simulink model "graphicalFun1"  (R2017b)
settings: Solver=FixedStepDiscrete  StartTime=0.0  StopTime=10.0  FixedStep=1  RelTol=1e-3
model workspace (MAT data in the model file):
  ContractValidatorBlocksMap = containers.Map
  ContractValidatorBlocksMap.serialization.keys = {'bacteriaPopulationStateflow/bacteriaPopulationSpec/validator', 'bacteriaPopulationStateflow1/bacteriaPopulationSpec/validator', 'bacteriaPopulationTruthTable/bacteriaPopulationSpec/validator', 'truthTable1/bacteriaPopulationSpec/validator', 'truthTable1_PP/bacteriaPopulationSpec/validator'}
  ContractValidatorBlocksMap.serialization.values{1}.block = 'bacteriaPopulationStateflow/bacteriaPopulationSpec/validator'
  ContractValidatorBlocksMap.serialization.values{1}.assumePorts = 1
  ContractValidatorBlocksMap.serialization.values{1}.guaranteePorts = 4
  ContractValidatorBlocksMap.serialization.values{1}.modeBlocksPorts = 3
  ContractValidatorBlocksMap.serialization.values{1}.portHandles.Inport = [317.001098633 318.000366211 319.000366211 320.000366211 321.000366211 322.000366211 323.000366211 324.000366211]
  ContractValidatorBlocksMap.serialization.values{1}.portHandles.Outport = 325.000366211
  ContractValidatorBlocksMap.serialization.values{1}.portHandles.Enable = []
  ContractValidatorBlocksMap.serialization.values{1}.portHandles.Trigger = []
  ContractValidatorBlocksMap.serialization.values{1}.portHandles.State = []
  ContractValidatorBlocksMap.serialization.values{1}.portHandles.LConn = []
  ContractValidatorBlocksMap.serialization.values{1}.portHandles.RConn = []
  ContractValidatorBlocksMap.serialization.values{1}.portHandles.Ifaction = []
  ContractValidatorBlocksMap.serialization.values{1}.portHandles.Reset = []
  ContractValidatorBlocksMap.serialization.values{1}.portConnectivity(1).Type = '1'
  ContractValidatorBlocksMap.serialization.values{1}.portConnectivity(1).Position = [360 -280]
  ContractValidatorBlocksMap.serialization.values{1}.portConnectivity(1).SrcBlock = 21.0003662109
  ContractValidatorBlocksMap.serialization.values{1}.portConnectivity(1).SrcPort = 0
  ContractValidatorBlocksMap.serialization.values{1}.portConnectivity(1).DstBlock = []
  ContractValidatorBlocksMap.serialization.values{1}.portConnectivity(1).DstPort = []
  ContractValidatorBlocksMap.serialization.values{1}.portConnectivity(2).Type = '2'
  ContractValidatorBlocksMap.serialization.values{1}.portConnectivity(2).Position = [360 -170]
  ContractValidatorBlocksMap.serialization.values{1}.portConnectivity(2).SrcBlock = 81.0003662109
  ContractValidatorBlocksMap.serialization.values{1}.portConnectivity(2).SrcPort = 0
  ContractValidatorBlocksMap.serialization.values{1}.portConnectivity(2).DstBlock = []
  ContractValidatorBlocksMap.serialization.values{1}.portConnectivity(2).DstPort = []
  ContractValidatorBlocksMap.serialization.values{1}.portConnectivity(3).Type = '3'
  ContractValidatorBlocksMap.serialization.values{1}.portConnectivity(3).Position = [360 -60]
  ContractValidatorBlocksMap.serialization.values{1}.portConnectivity(3).SrcBlock = 87.0010986328
  ContractValidatorBlocksMap.serialization.values{1}.portConnectivity(3).SrcPort = 0
  ContractValidatorBlocksMap.serialization.values{1}.portConnectivity(3).DstBlock = []
  ContractValidatorBlocksMap.serialization.values{1}.portConnectivity(3).DstPort = []
  ContractValidatorBlocksMap.serialization.values{1}.portConnectivity(4).Type = '4'
  ContractValidatorBlocksMap.serialization.values{1}.portConnectivity(4).Position = [360 50]
  ContractValidatorBlocksMap.serialization.values{1}.portConnectivity(4).SrcBlock = 99.0010986328
  ContractValidatorBlocksMap.serialization.values{1}.portConnectivity(4).SrcPort = 0
  ContractValidatorBlocksMap.serialization.values{1}.portConnectivity(4).DstBlock = []
  ContractValidatorBlocksMap.serialization.values{1}.portConnectivity(4).DstPort = []
  ContractValidatorBlocksMap.serialization.values{1}.portConnectivity(5).Type = '5'
  ContractValidatorBlocksMap.serialization.values{1}.portConnectivity(5).Position = [360 160]
  ContractValidatorBlocksMap.serialization.values{1}.portConnectivity(5).SrcBlock = 148.001098633
  ContractValidatorBlocksMap.serialization.values{1}.portConnectivity(5).SrcPort = 0
  ContractValidatorBlocksMap.serialization.values{1}.portConnectivity(5).DstBlock = []
  ContractValidatorBlocksMap.serialization.values{1}.portConnectivity(5).DstPort = []
  ContractValidatorBlocksMap.serialization.values{1}.portConnectivity(6).Type = '6'
  ContractValidatorBlocksMap.serialization.values{1}.portConnectivity(6).Position = [360 270]
  ContractValidatorBlocksMap.serialization.values{1}.portConnectivity(6).SrcBlock = 197.001098633
  ContractValidatorBlocksMap.serialization.values{1}.portConnectivity(6).SrcPort = 0
  ContractValidatorBlocksMap.serialization.values{1}.portConnectivity(6).DstBlock = []
  ContractValidatorBlocksMap.serialization.values{1}.portConnectivity(6).DstPort = []
  ContractValidatorBlocksMap.serialization.values{1}.portConnectivity(7).Type = '7'
  ContractValidatorBlocksMap.serialization.values{1}.portConnectivity(7).Position = [360 380]
  ContractValidatorBlocksMap.serialization.values{1}.portConnectivity(7).SrcBlock = 27.0010986328
  ContractValidatorBlocksMap.serialization.values{1}.portConnectivity(7).SrcPort = 0
  ContractValidatorBlocksMap.serialization.values{1}.portConnectivity(7).DstBlock = []
  ContractValidatorBlocksMap.serialization.values{1}.portConnectivity(7).DstPort = []
  ContractValidatorBlocksMap.serialization.values{1}.portConnectivity(8).Type = '8'
  ContractValidatorBlocksMap.serialization.values{1}.portConnectivity(8).Position = [360 490]
  ContractValidatorBlocksMap.serialization.values{1}.portConnectivity(8).SrcBlock = 238.001098633
  ContractValidatorBlocksMap.serialization.values{1}.portConnectivity(8).SrcPort = 0
  ContractValidatorBlocksMap.serialization.values{1}.portConnectivity(8).DstBlock = []
  ContractValidatorBlocksMap.serialization.values{1}.portConnectivity(8).DstPort = []
  ContractValidatorBlocksMap.serialization.values{1}.portConnectivity(9).Type = '1'
  ContractValidatorBlocksMap.serialization.values{1}.portConnectivity(9).Position = [500 105]
  ContractValidatorBlocksMap.serialization.values{1}.portConnectivity(9).SrcBlock = []
  ContractValidatorBlocksMap.serialization.values{1}.portConnectivity(9).SrcPort = []
  ContractValidatorBlocksMap.serialization.values{1}.portConnectivity(9).DstBlock = [250.000366211 20.0003662109]
  ContractValidatorBlocksMap.serialization.values{1}.portConnectivity(9).DstPort = [0 0]
  ContractValidatorBlocksMap.serialization.values{2}.block = 'bacteriaPopulationStateflow1/bacteriaPopulationSpec/validator'
  ContractValidatorBlocksMap.serialization.values{2}.assumePorts = 1
  ContractValidatorBlocksMap.serialization.values{2}.guaranteePorts = 4
  ContractValidatorBlocksMap.serialization.values{2}.modeBlocksPorts = 3
  ContractValidatorBlocksMap.serialization.values{2}.portHandles.Inport = [309.001586914 310.001220703 311.000854492 312.000976562 313.000976562 314.001098633 315.000976562 316.000854492]
  ContractValidatorBlocksMap.serialization.values{2}.portHandles.Outport = 317.001098633
  ContractValidatorBlocksMap.serialization.values{2}.portHandles.Enable = []
  ContractValidatorBlocksMap.serialization.values{2}.portHandles.Trigger = []
  ContractValidatorBlocksMap.serialization.values{2}.portHandles.State = []
  ContractValidatorBlocksMap.serialization.values{2}.portHandles.LConn = []
  ContractValidatorBlocksMap.serialization.values{2}.portHandles.RConn = []
  ContractValidatorBlocksMap.serialization.values{2}.portHandles.Ifaction = []
  ContractValidatorBlocksMap.serialization.values{2}.portHandles.Reset = []
  ContractValidatorBlocksMap.serialization.values{2}.portConnectivity(1).Type = '1'
  ContractValidatorBlocksMap.serialization.values{2}.portConnectivity(1).Position = [360 -280]
  ContractValidatorBlocksMap.serialization.values{2}.portConnectivity(1).SrcBlock = 21.0007324219
  ContractValidatorBlocksMap.serialization.values{2}.portConnectivity(1).SrcPort = 0
  ContractValidatorBlocksMap.serialization.values{2}.portConnectivity(1).DstBlock = []
  ContractValidatorBlocksMap.serialization.values{2}.portConnectivity(1).DstPort = []
  ContractValidatorBlocksMap.serialization.values{2}.portConnectivity(2).Type = '2'
  ContractValidatorBlocksMap.serialization.values{2}.portConnectivity(2).Position = [360 -170]
  ContractValidatorBlocksMap.serialization.values{2}.portConnectivity(2).SrcBlock = 81.0010986328
  ContractValidatorBlocksMap.serialization.values{2}.portConnectivity(2).SrcPort = 0
  ContractValidatorBlocksMap.serialization.values{2}.portConnectivity(2).DstBlock = []
  ContractValidatorBlocksMap.serialization.values{2}.portConnectivity(2).DstPort = []
  ContractValidatorBlocksMap.serialization.values{2}.portConnectivity(3).Type = '3'
  ContractValidatorBlocksMap.serialization.values{2}.portConnectivity(3).Position = [360 -60]
  ContractValidatorBlocksMap.serialization.values{2}.portConnectivity(3).SrcBlock = 87.0009765625
  ContractValidatorBlocksMap.serialization.values{2}.portConnectivity(3).SrcPort = 0
  ContractValidatorBlocksMap.serialization.values{2}.portConnectivity(3).DstBlock = []
  ContractValidatorBlocksMap.serialization.values{2}.portConnectivity(3).DstPort = []
  ContractValidatorBlocksMap.serialization.values{2}.portConnectivity(4).Type = '4'
  ContractValidatorBlocksMap.serialization.values{2}.portConnectivity(4).Position = [360 50]
  ContractValidatorBlocksMap.serialization.values{2}.portConnectivity(4).SrcBlock = 99.0009765625
  ContractValidatorBlocksMap.serialization.values{2}.portConnectivity(4).SrcPort = 0
  ContractValidatorBlocksMap.serialization.values{2}.portConnectivity(4).DstBlock = []
  ContractValidatorBlocksMap.serialization.values{2}.portConnectivity(4).DstPort = []
  ContractValidatorBlocksMap.serialization.values{2}.portConnectivity(5).Type = '5'
  ContractValidatorBlocksMap.serialization.values{2}.portConnectivity(5).Position = [360 160]
  ContractValidatorBlocksMap.serialization.values{2}.portConnectivity(5).SrcBlock = 148.000976562
  ContractValidatorBlocksMap.serialization.values{2}.portConnectivity(5).SrcPort = 0
  ContractValidatorBlocksMap.serialization.values{2}.portConnectivity(5).DstBlock = []
  ContractValidatorBlocksMap.serialization.values{2}.portConnectivity(5).DstPort = []
  ContractValidatorBlocksMap.serialization.values{2}.portConnectivity(6).Type = '6'
  ContractValidatorBlocksMap.serialization.values{2}.portConnectivity(6).Position = [360 270]
  ContractValidatorBlocksMap.serialization.values{2}.portConnectivity(6).SrcBlock = 197.000976562
  ContractValidatorBlocksMap.serialization.values{2}.portConnectivity(6).SrcPort = 0
  ContractValidatorBlocksMap.serialization.values{2}.portConnectivity(6).DstBlock = []
  ContractValidatorBlocksMap.serialization.values{2}.portConnectivity(6).DstPort = []
  ContractValidatorBlocksMap.serialization.values{2}.portConnectivity(7).Type = '7'
  ContractValidatorBlocksMap.serialization.values{2}.portConnectivity(7).Position = [360 380]
  ContractValidatorBlocksMap.serialization.values{2}.portConnectivity(7).SrcBlock = 27.0018310547
  ContractValidatorBlocksMap.serialization.values{2}.portConnectivity(7).SrcPort = 0
  ContractValidatorBlocksMap.serialization.values{2}.portConnectivity(7).DstBlock = []
  ContractValidatorBlocksMap.serialization.values{2}.portConnectivity(7).DstPort = []
  ContractValidatorBlocksMap.serialization.values{2}.portConnectivity(8).Type = '8'
  ContractValidatorBlocksMap.serialization.values{2}.portConnectivity(8).Position = [360 490]
  ContractValidatorBlocksMap.serialization.values{2}.portConnectivity(8).SrcBlock = 238.000976562
  ContractValidatorBlocksMap.serialization.values{2}.portConnectivity(8).SrcPort = 0
  ContractValidatorBlocksMap.serialization.values{2}.portConnectivity(8).DstBlock = []
  ContractValidatorBlocksMap.serialization.values{2}.portConnectivity(8).DstPort = []
  ContractValidatorBlocksMap.serialization.values{2}.portConnectivity(9).Type = '1'
  ContractValidatorBlocksMap.serialization.values{2}.portConnectivity(9).Position = [500 105]
  ContractValidatorBlocksMap.serialization.values{2}.portConnectivity(9).SrcBlock = []
  ContractValidatorBlocksMap.serialization.values{2}.portConnectivity(9).SrcPort = []
  ContractValidatorBlocksMap.serialization.values{2}.portConnectivity(9).DstBlock = [250.000488281 20.0009765625]
  ContractValidatorBlocksMap.serialization.values{2}.portConnectivity(9).DstPort = [0 0]
  ContractValidatorBlocksMap.serialization.values{3}.block = 'bacteriaPopulationTruthTable/bacteriaPopulationSpec/validator'
  ContractValidatorBlocksMap.serialization.values{3}.assumePorts = 1
  ContractValidatorBlocksMap.serialization.values{3}.guaranteePorts = 4
  ContractValidatorBlocksMap.serialization.values{3}.modeBlocksPorts = 3
  ContractValidatorBlocksMap.serialization.values{3}.portHandles.Inport = [317.001831055 318.001342773 319.001342773 320.001342773 321.001342773 322.001342773 323.001342773 324.001342773]
  ContractValidatorBlocksMap.serialization.values{3}.portHandles.Outport = 325.000976562
  ContractValidatorBlocksMap.serialization.values{3}.portHandles.Enable = []
  ContractValidatorBlocksMap.serialization.values{3}.portHandles.Trigger = []
  ContractValidatorBlocksMap.serialization.values{3}.portHandles.State = []
  ContractValidatorBlocksMap.serialization.values{3}.portHandles.LConn = []
  ContractValidatorBlocksMap.serialization.values{3}.portHandles.RConn = []
  ContractValidatorBlocksMap.serialization.values{3}.portHandles.Ifaction = []
  ContractValidatorBlocksMap.serialization.values{3}.portHandles.Reset = []
  ContractValidatorBlocksMap.serialization.values{3}.portConnectivity(1).Type = '1'
  ContractValidatorBlocksMap.serialization.values{3}.portConnectivity(1).Position = [360 -280]
  ContractValidatorBlocksMap.serialization.values{3}.portConnectivity(1).SrcBlock = 21.0007324219
  ContractValidatorBlocksMap.serialization.values{3}.portConnectivity(1).SrcPort = 0
  ContractValidatorBlocksMap.serialization.values{3}.portConnectivity(1).DstBlock = []
  ContractValidatorBlocksMap.serialization.values{3}.portConnectivity(1).DstPort = []
  ContractValidatorBlocksMap.serialization.values{3}.portConnectivity(2).Type = '2'
  ContractValidatorBlocksMap.serialization.values{3}.portConnectivity(2).Position = [360 -170]
  ContractValidatorBlocksMap.serialization.values{3}.portConnectivity(2).SrcBlock = 81.0007324219
  ContractValidatorBlocksMap.serialization.values{3}.portConnectivity(2).SrcPort = 0
  ContractValidatorBlocksMap.serialization.values{3}.portConnectivity(2).DstBlock = []
  ContractValidatorBlocksMap.serialization.values{3}.portConnectivity(2).DstPort = []
  ContractValidatorBlocksMap.serialization.values{3}.portConnectivity(3).Type = '3'
  ContractValidatorBlocksMap.serialization.values{3}.portConnectivity(3).Position = [360 -60]
  ContractValidatorBlocksMap.serialization.values{3}.portConnectivity(3).SrcBlock = 87.0012207031
  ContractValidatorBlocksMap.serialization.values{3}.portConnectivity(3).SrcPort = 0
  ContractValidatorBlocksMap.serialization.values{3}.portConnectivity(3).DstBlock = []
  ContractValidatorBlocksMap.serialization.values{3}.portConnectivity(3).DstPort = []
  ContractValidatorBlocksMap.serialization.values{3}.portConnectivity(4).Type = '4'
  ContractValidatorBlocksMap.serialization.values{3}.portConnectivity(4).Position = [360 50]
  ContractValidatorBlocksMap.serialization.values{3}.portConnectivity(4).SrcBlock = 99.0014648438
  ContractValidatorBlocksMap.serialization.values{3}.portConnectivity(4).SrcPort = 0
  ContractValidatorBlocksMap.serialization.values{3}.portConnectivity(4).DstBlock = []
  ContractValidatorBlocksMap.serialization.values{3}.portConnectivity(4).DstPort = []
  ContractValidatorBlocksMap.serialization.values{3}.portConnectivity(5).Type = '5'
  ContractValidatorBlocksMap.serialization.values{3}.portConnectivity(5).Position = [360 160]
  ContractValidatorBlocksMap.serialization.values{3}.portConnectivity(5).SrcBlock = 148.001220703
  ContractValidatorBlocksMap.serialization.values{3}.portConnectivity(5).SrcPort = 0
  ContractValidatorBlocksMap.serialization.values{3}.portConnectivity(5).DstBlock = []
  ContractValidatorBlocksMap.serialization.values{3}.portConnectivity(5).DstPort = []
  ContractValidatorBlocksMap.serialization.values{3}.portConnectivity(6).Type = '6'
  ContractValidatorBlocksMap.serialization.values{3}.portConnectivity(6).Position = [360 270]
  ContractValidatorBlocksMap.serialization.values{3}.portConnectivity(6).SrcBlock = 197.001098633
  ContractValidatorBlocksMap.serialization.values{3}.portConnectivity(6).SrcPort = 0
  ContractValidatorBlocksMap.serialization.values{3}.portConnectivity(6).DstBlock = []
  ContractValidatorBlocksMap.serialization.values{3}.portConnectivity(6).DstPort = []
  ContractValidatorBlocksMap.serialization.values{3}.portConnectivity(7).Type = '7'
  ContractValidatorBlocksMap.serialization.values{3}.portConnectivity(7).Position = [360 380]
  ContractValidatorBlocksMap.serialization.values{3}.portConnectivity(7).SrcBlock = 27.0021972656
  ContractValidatorBlocksMap.serialization.values{3}.portConnectivity(7).SrcPort = 0
  ContractValidatorBlocksMap.serialization.values{3}.portConnectivity(7).DstBlock = []
  ContractValidatorBlocksMap.serialization.values{3}.portConnectivity(7).DstPort = []
  ContractValidatorBlocksMap.serialization.values{3}.portConnectivity(8).Type = '8'
  ContractValidatorBlocksMap.serialization.values{3}.portConnectivity(8).Position = [360 490]
  ContractValidatorBlocksMap.serialization.values{3}.portConnectivity(8).SrcBlock = 238.001098633
  ContractValidatorBlocksMap.serialization.values{3}.portConnectivity(8).SrcPort = 0
  ContractValidatorBlocksMap.serialization.values{3}.portConnectivity(8).DstBlock = []
  ContractValidatorBlocksMap.serialization.values{3}.portConnectivity(8).DstPort = []
  ContractValidatorBlocksMap.serialization.values{3}.portConnectivity(9).Type = '1'
  ContractValidatorBlocksMap.serialization.values{3}.portConnectivity(9).Position = [500 105]
  ContractValidatorBlocksMap.serialization.values{3}.portConnectivity(9).SrcBlock = []
  ContractValidatorBlocksMap.serialization.values{3}.portConnectivity(9).SrcPort = []
  ContractValidatorBlocksMap.serialization.values{3}.portConnectivity(9).DstBlock = [250.000610352 20.0007324219]
  ContractValidatorBlocksMap.serialization.values{3}.portConnectivity(9).DstPort = [0 0]
  ContractValidatorBlocksMap.serialization.values{4}.block = 'truthTable1/bacteriaPopulationSpec/validator'
  ContractValidatorBlocksMap.serialization.values{4}.assumePorts = 1
  ContractValidatorBlocksMap.serialization.values{4}.guaranteePorts = 4
  ContractValidatorBlocksMap.serialization.values{4}.modeBlocksPorts = 3
  ContractValidatorBlocksMap.serialization.values{4}.portHandles.Inport = [317.000732422 318.000244141 319.000244141 320.000244141 321.000244141 322.000244141 323.000244141 324.000244141]
  ContractValidatorBlocksMap.serialization.values{4}.portHandles.Outport = 325.000244141
  ContractValidatorBlocksMap.serialization.values{4}.portHandles.Enable = []
  ContractValidatorBlocksMap.serialization.values{4}.portHandles.Trigger = []
  ContractValidatorBlocksMap.serialization.values{4}.portHandles.State = []
  ContractValidatorBlocksMap.serialization.values{4}.portHandles.LConn = []
  ContractValidatorBlocksMap.serialization.values{4}.portHandles.RConn = []
  ContractValidatorBlocksMap.serialization.values{4}.portHandles.Ifaction = []
  ContractValidatorBlocksMap.serialization.values{4}.portHandles.Reset = []
  ContractValidatorBlocksMap.serialization.values{4}.portConnectivity(1).Type = '1'
  ContractValidatorBlocksMap.serialization.values{4}.portConnectivity(1).Position = [360 -280]
  ContractValidatorBlocksMap.serialization.values{4}.portConnectivity(1).SrcBlock = 21.0002441406
  ContractValidatorBlocksMap.serialization.values{4}.portConnectivity(1).SrcPort = 0
  ContractValidatorBlocksMap.serialization.values{4}.portConnectivity(1).DstBlock = []
  ContractValidatorBlocksMap.serialization.values{4}.portConnectivity(1).DstPort = []
  ContractValidatorBlocksMap.serialization.values{4}.portConnectivity(2).Type = '2'
  ContractValidatorBlocksMap.serialization.values{4}.portConnectivity(2).Position = [360 -170]
  ContractValidatorBlocksMap.serialization.values{4}.portConnectivity(2).SrcBlock = 81.0002441406
  ContractValidatorBlocksMap.serialization.values{4}.portConnectivity(2).SrcPort = 0
  ContractValidatorBlocksMap.serialization.values{4}.portConnectivity(2).DstBlock = []
  ContractValidatorBlocksMap.serialization.values{4}.portConnectivity(2).DstPort = []
  ContractValidatorBlocksMap.serialization.values{4}.portConnectivity(3).Type = '3'
  ContractValidatorBlocksMap.serialization.values{4}.portConnectivity(3).Position = [360 -60]
  ContractValidatorBlocksMap.serialization.values{4}.portConnectivity(3).SrcBlock = 87.0007324219
  ContractValidatorBlocksMap.serialization.values{4}.portConnectivity(3).SrcPort = 0
  ContractValidatorBlocksMap.serialization.values{4}.portConnectivity(3).DstBlock = []
  ContractValidatorBlocksMap.serialization.values{4}.portConnectivity(3).DstPort = []
  ContractValidatorBlocksMap.serialization.values{4}.portConnectivity(4).Type = '4'
  ContractValidatorBlocksMap.serialization.values{4}.portConnectivity(4).Position = [360 50]
  ContractValidatorBlocksMap.serialization.values{4}.portConnectivity(4).SrcBlock = 99.0007324219
  ContractValidatorBlocksMap.serialization.values{4}.portConnectivity(4).SrcPort = 0
  ContractValidatorBlocksMap.serialization.values{4}.portConnectivity(4).DstBlock = []
  ContractValidatorBlocksMap.serialization.values{4}.portConnectivity(4).DstPort = []
  ContractValidatorBlocksMap.serialization.values{4}.portConnectivity(5).Type = '5'
  ContractValidatorBlocksMap.serialization.values{4}.portConnectivity(5).Position = [360 160]
  ContractValidatorBlocksMap.serialization.values{4}.portConnectivity(5).SrcBlock = 148.000732422
  ContractValidatorBlocksMap.serialization.values{4}.portConnectivity(5).SrcPort = 0
  ContractValidatorBlocksMap.serialization.values{4}.portConnectivity(5).DstBlock = []
  ContractValidatorBlocksMap.serialization.values{4}.portConnectivity(5).DstPort = []
  ContractValidatorBlocksMap.serialization.values{4}.portConnectivity(6).Type = '6'
  ContractValidatorBlocksMap.serialization.values{4}.portConnectivity(6).Position = [360 270]
  ContractValidatorBlocksMap.serialization.values{4}.portConnectivity(6).SrcBlock = 197.000732422
  ContractValidatorBlocksMap.serialization.values{4}.portConnectivity(6).SrcPort = 0
  ContractValidatorBlocksMap.serialization.values{4}.portConnectivity(6).DstBlock = []
  ContractValidatorBlocksMap.serialization.values{4}.portConnectivity(6).DstPort = []
  ContractValidatorBlocksMap.serialization.values{4}.portConnectivity(7).Type = '7'
  ContractValidatorBlocksMap.serialization.values{4}.portConnectivity(7).Position = [360 380]
  ContractValidatorBlocksMap.serialization.values{4}.portConnectivity(7).SrcBlock = 27.0007324219
  ContractValidatorBlocksMap.serialization.values{4}.portConnectivity(7).SrcPort = 0
  ContractValidatorBlocksMap.serialization.values{4}.portConnectivity(7).DstBlock = []
  ContractValidatorBlocksMap.serialization.values{4}.portConnectivity(7).DstPort = []
  ContractValidatorBlocksMap.serialization.values{4}.portConnectivity(8).Type = '8'
  ContractValidatorBlocksMap.serialization.values{4}.portConnectivity(8).Position = [360 490]
  ContractValidatorBlocksMap.serialization.values{4}.portConnectivity(8).SrcBlock = 238.000732422
  ContractValidatorBlocksMap.serialization.values{4}.portConnectivity(8).SrcPort = 0
  ContractValidatorBlocksMap.serialization.values{4}.portConnectivity(8).DstBlock = []
  ContractValidatorBlocksMap.serialization.values{4}.portConnectivity(8).DstPort = []
  ContractValidatorBlocksMap.serialization.values{4}.portConnectivity(9).Type = '1'
  ContractValidatorBlocksMap.serialization.values{4}.portConnectivity(9).Position = [500 105]
  ContractValidatorBlocksMap.serialization.values{4}.portConnectivity(9).SrcBlock = []
  ContractValidatorBlocksMap.serialization.values{4}.portConnectivity(9).SrcPort = []
  ContractValidatorBlocksMap.serialization.values{4}.portConnectivity(9).DstBlock = [250.000244141 20.0002441406]
  ContractValidatorBlocksMap.serialization.values{4}.portConnectivity(9).DstPort = [0 0]
  ContractValidatorBlocksMap.serialization.values{5}.block = 'truthTable1_PP/bacteriaPopulationSpec/validator'
  ContractValidatorBlocksMap.serialization.values{5}.assumePorts = 1
  ContractValidatorBlocksMap.serialization.values{5}.guaranteePorts = 4
  ContractValidatorBlocksMap.serialization.values{5}.modeBlocksPorts = 3
  ContractValidatorBlocksMap.serialization.values{5}.portHandles.Inport = [1295.00036621 1296.00012207 1297.00012207 1298.00012207 1299.00012207 1300.00012207 1301.00012207 1302.00012207]
  ContractValidatorBlocksMap.serialization.values{5}.portHandles.Outport = 1303.00012207
  ContractValidatorBlocksMap.serialization.values{5}.portHandles.Enable = []
  ContractValidatorBlocksMap.serialization.values{5}.portHandles.Trigger = []
  ContractValidatorBlocksMap.serialization.values{5}.portHandles.State = []
  ContractValidatorBlocksMap.serialization.values{5}.portHandles.LConn = []
  ContractValidatorBlocksMap.serialization.values{5}.portHandles.RConn = []
  ContractValidatorBlocksMap.serialization.values{5}.portHandles.Ifaction = []
  ContractValidatorBlocksMap.serialization.values{5}.portHandles.Reset = []
  ContractValidatorBlocksMap.serialization.values{5}.portConnectivity(1).Type = '1'
  ContractValidatorBlocksMap.serialization.values{5}.portConnectivity(1).Position = [360 -280]
  ContractValidatorBlocksMap.serialization.values{5}.portConnectivity(1).SrcBlock = 350.000488281
  ContractValidatorBlocksMap.serialization.values{5}.portConnectivity(1).SrcPort = 0
  ContractValidatorBlocksMap.serialization.values{5}.portConnectivity(1).DstBlock = []
  ContractValidatorBlocksMap.serialization.values{5}.portConnectivity(1).DstPort = []
  ContractValidatorBlocksMap.serialization.values{5}.portConnectivity(2).Type = '2'
  ContractValidatorBlocksMap.serialization.values{5}.portConnectivity(2).Position = [360 -170]
  ContractValidatorBlocksMap.serialization.values{5}.portConnectivity(2).SrcBlock = 419.000488281
  ContractValidatorBlocksMap.serialization.values{5}.portConnectivity(2).SrcPort = 0
  ContractValidatorBlocksMap.serialization.values{5}.portConnectivity(2).DstBlock = []
  ContractValidatorBlocksMap.serialization.values{5}.portConnectivity(2).DstPort = []
  ContractValidatorBlocksMap.serialization.values{5}.portConnectivity(3).Type = '3'
  ContractValidatorBlocksMap.serialization.values{5}.portConnectivity(3).Position = [360 -60]
  ContractValidatorBlocksMap.serialization.values{5}.portConnectivity(3).SrcBlock = 425.000488281
  ContractValidatorBlocksMap.serialization.values{5}.portConnectivity(3).SrcPort = 0
  ContractValidatorBlocksMap.serialization.values{5}.portConnectivity(3).DstBlock = []
  ContractValidatorBlocksMap.serialization.values{5}.portConnectivity(3).DstPort = []
  ContractValidatorBlocksMap.serialization.values{5}.portConnectivity(4).Type = '4'
  ContractValidatorBlocksMap.serialization.values{5}.portConnectivity(4).Position = [360 50]
  ContractValidatorBlocksMap.serialization.values{5}.portConnectivity(4).SrcBlock = 437.000488281
  ContractValidatorBlocksMap.serialization.values{5}.portConnectivity(4).SrcPort = 0
  ContractValidatorBlocksMap.serialization.values{5}.portConnectivity(4).DstBlock = []
  ContractValidatorBlocksMap.serialization.values{5}.portConnectivity(4).DstPort = []
  ContractValidatorBlocksMap.serialization.values{5}.portConnectivity(5).Type = '5'
  ContractValidatorBlocksMap.serialization.values{5}.portConnectivity(5).Position = [360 160]
  ContractValidatorBlocksMap.serialization.values{5}.portConnectivity(5).SrcBlock = 1134.00036621
  ContractValidatorBlocksMap.serialization.values{5}.portConnectivity(5).SrcPort = 0
  ContractValidatorBlocksMap.serialization.values{5}.portConnectivity(5).DstBlock = []
  ContractValidatorBlocksMap.serialization.values{5}.portConnectivity(5).DstPort = []
  ContractValidatorBlocksMap.serialization.values{5}.portConnectivity(6).Type = '6'
  ContractValidatorBlocksMap.serialization.values{5}.portConnectivity(6).Position = [360 270]
  ContractValidatorBlocksMap.serialization.values{5}.portConnectivity(6).SrcBlock = 1183.00036621
  ContractValidatorBlocksMap.serialization.values{5}.portConnectivity(6).SrcPort = 0
  ContractValidatorBlocksMap.serialization.values{5}.portConnectivity(6).DstBlock = []
  ContractValidatorBlocksMap.serialization.values{5}.portConnectivity(6).DstPort = []
  ContractValidatorBlocksMap.serialization.values{5}.portConnectivity(7).Type = '7'
  ContractValidatorBlocksMap.serialization.values{5}.portConnectivity(7).Position = [360 380]
  ContractValidatorBlocksMap.serialization.values{5}.portConnectivity(7).SrcBlock = 356.001464844
  ContractValidatorBlocksMap.serialization.values{5}.portConnectivity(7).SrcPort = 0
  ContractValidatorBlocksMap.serialization.values{5}.portConnectivity(7).DstBlock = []
  ContractValidatorBlocksMap.serialization.values{5}.portConnectivity(7).DstPort = []
  ContractValidatorBlocksMap.serialization.values{5}.portConnectivity(8).Type = '8'
  ContractValidatorBlocksMap.serialization.values{5}.portConnectivity(8).Position = [360 490]
  ContractValidatorBlocksMap.serialization.values{5}.portConnectivity(8).SrcBlock = 1224.00036621
  ContractValidatorBlocksMap.serialization.values{5}.portConnectivity(8).SrcPort = 0
  ContractValidatorBlocksMap.serialization.values{5}.portConnectivity(8).DstBlock = []
  ContractValidatorBlocksMap.serialization.values{5}.portConnectivity(8).DstPort = []
  ContractValidatorBlocksMap.serialization.values{5}.portConnectivity(9).Type = '1'
  ContractValidatorBlocksMap.serialization.values{5}.portConnectivity(9).Position = [500 105]
  ContractValidatorBlocksMap.serialization.values{5}.portConnectivity(9).SrcBlock = []
  ContractValidatorBlocksMap.serialization.values{5}.portConnectivity(9).SrcPort = []
  ContractValidatorBlocksMap.serialization.values{5}.portConnectivity(9).DstBlock = [1236.00012207 349.000488281]
  ContractValidatorBlocksMap.serialization.values{5}.portConnectivity(9).DstPort = [0 0]
  ContractValidatorBlocksMap.serialization.uniformity = 0
  ContractValidatorBlocksMap.serialization.keyType = 'char'
  ContractValidatorBlocksMap.serialization.valueType = 'any'
  already_pp = 1
undefined symbols (not defined in the file): ArrowOperator, contractAfterSimulation, ContractAssumeBlock, contractBeforeSimulation, ContractBlock, ContractEnsureBlock, ContractGuaranteeBlock, ContractModeBlock, ContractRequireBlock, ContractValidatorBlock, saveValidatorParameters
settings Model: Creator=Mudathir  LastModifiedBy=hbourbou
settings OptimizationCC: LifeSpan=inf
settings DebuggingCC: AlgebraicLoopMsg=error  SFExecutionAtInitializationDiag=none
settings HardwareCC: ProdBitPerSizeT=32  ProdBitPerPtrDiffT=32  ProdWordSize=32  ProdHWDeviceType=Specified
settings CodeAppCC: StateflowObjectComments=on

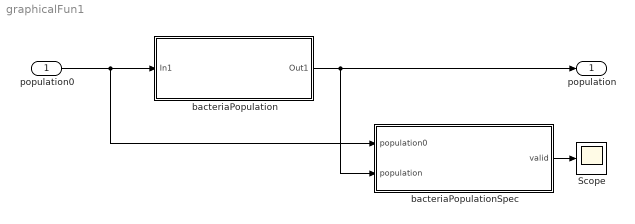
== system graphicalFun1 ==
  population0 : Inport
  Scope : Scope
  bacteriaPopulation : Subsystem  TreatAsAtomicUnit=on
  bacteriaPopulationSpec : Subsystem  TreatAsAtomicUnit=on  mask(ContractBlock){ContractBlockType=ContractBlock}
      mask init:
      | set_param(gcb, 'LinkStatus', 'none');
      mask DialogControl DescTextVar Prompt: Contract block
      mask Display:
      | text(0.5, 0.5, '{\bf\fontsize{20}Contract}', 'hor', 'center', 'texmode','on');
      | blocks = find_system(gcb, 'LookUnderMasks','all', 'SearchDepth',1,'BlockType','Inport');
      | for i = 1 : length(blocks)
      |     blockName = get_param(blocks(i), 'Name');
      |     [path, blockName] = fileparts(char(blockName));
      |     port_label('input', i, blockName);
      | end
      | 
      | blocks = find_system(gcb, 'LookUnderMasks','all', 'SearchDepth',1,'BlockType','Outport');
      | for i = 1 : length(blocks)
      |     blockName = get_param(blocks(i), 'Name');
      |     [path, blockName] = fileparts(char(blockName));
      |     port_label('output', i, blockName);
      | end
  population : Outport
  wires:
  population0/1 -> bacteriaPopulation/1(In1), bacteriaPopulationSpec/1(population0)
  bacteriaPopulationSpec/1(valid) -> Scope/1
  bacteriaPopulation/1(Out1) -> bacteriaPopulationSpec/2(population), population/1

== system graphicalFun1/bacteriaPopulation ==
  In1 : Inport
  bacteriaPopulation : Stateflow chart  TreatAsAtomicUnit=on
  Out1 : Outport
  wires:
  bacteriaPopulation/1(population) -> Out1/1
  In1/1 -> bacteriaPopulation/1(population0)

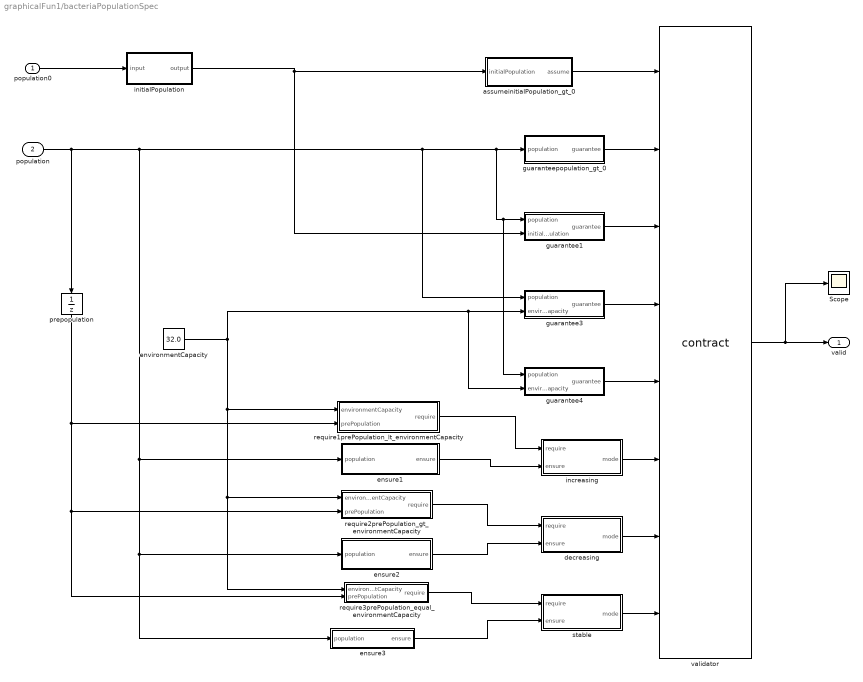
== system graphicalFun1/bacteriaPopulationSpec ==
  population0 : Inport
  population : Inport  Port=2
  Scope : Scope
  assumeinitialPopulation_gt_0 : Subsystem  TreatAsAtomicUnit=on  mask(ContractAssumeBlock){ContractBlockType=ContractAssumeBlock}
      mask init:
      | set_param(gcb, 'LinkStatus', 'none');
      mask DialogControl DescTextVar Prompt: Assume block
  decreasing : Subsystem  TreatAsAtomicUnit=on  mask(ContractModeBlock){ContractBlockType=ContractModeBlock}
      mask init:
      | set_param(gcb, 'LinkStatus', 'none');
      mask DialogControl DescTextVar Prompt: Mode block
  ensure1 : Subsystem  TreatAsAtomicUnit=on  mask(ContractEnsureBlock){ContractBlockType=ContractEnsureBlock}
      mask init:
      | set_param(gcb, 'LinkStatus', 'none');
      mask DialogControl DescTextVar Prompt: Ensure block
  ensure2 : Subsystem  TreatAsAtomicUnit=on  mask(ContractEnsureBlock){ContractBlockType=ContractEnsureBlock}
      mask init:
      | set_param(gcb, 'LinkStatus', 'none');
      mask DialogControl DescTextVar Prompt: Ensure block
  ensure3 : Subsystem  TreatAsAtomicUnit=on  mask(ContractEnsureBlock){ContractBlockType=ContractEnsureBlock}
      mask init:
      | set_param(gcb, 'LinkStatus', 'none');
      mask DialogControl DescTextVar Prompt: Ensure block
  environmentCapacity : Constant  Value=32.0  OutDataTypeStr=double
  guarantee1 : Subsystem  TreatAsAtomicUnit=on  mask(ContractGuaranteeBlock){ContractBlockType=ContractGuaranteeBlock}
      mask init:
      | set_param(gcb, 'LinkStatus', 'none');
      mask DialogControl DescTextVar Prompt: Guarantee block
  guarantee3 : Subsystem  TreatAsAtomicUnit=on  mask(ContractGuaranteeBlock){ContractBlockType=ContractGuaranteeBlock}
      mask init:
      | set_param(gcb, 'LinkStatus', 'none');
      mask DialogControl DescTextVar Prompt: Guarantee block
  guarantee4 : Subsystem  TreatAsAtomicUnit=on  mask(ContractGuaranteeBlock){ContractBlockType=ContractGuaranteeBlock}
      mask init:
      | set_param(gcb, 'LinkStatus', 'none');
      mask DialogControl DescTextVar Prompt: Guarantee block
  guaranteepopulation_gt_0 : Subsystem  TreatAsAtomicUnit=on  mask(ContractGuaranteeBlock){ContractBlockType=ContractGuaranteeBlock}
      mask init:
      | set_param(gcb, 'LinkStatus', 'none');
      mask DialogControl DescTextVar Prompt: Guarantee block
  increasing : Subsystem  TreatAsAtomicUnit=on  mask(ContractModeBlock){ContractBlockType=ContractModeBlock}
      mask init:
      | set_param(gcb, 'LinkStatus', 'none');
      mask DialogControl DescTextVar Prompt: Mode block
  initialPopulation : Subsystem  TreatAsAtomicUnit=on
  prepopulation : UnitDelay  SampleTime=-1
  require1prePopulation_lt_environmentCapacity : Subsystem  TreatAsAtomicUnit=on  mask(ContractRequireBlock){ContractBlockType=ContractRequireBlock}
      mask init:
      | set_param(gcb, 'LinkStatus', 'none');
      mask DialogControl DescTextVar Prompt: Require block
  require2prePopulation_gt_environmentCapacity : Subsystem  TreatAsAtomicUnit=on  mask(ContractRequireBlock){ContractBlockType=ContractRequireBlock}
      mask init:
      | set_param(gcb, 'LinkStatus', 'none');
      mask DialogControl DescTextVar Prompt: Require block
  require3prePopulation_equal_environmentCapacity : Subsystem  TreatAsAtomicUnit=on  mask(ContractRequireBlock){ContractBlockType=ContractRequireBlock}
      mask init:
      | set_param(gcb, 'LinkStatus', 'none');
      mask DialogControl DescTextVar Prompt: Require block
  stable : Subsystem  TreatAsAtomicUnit=on  mask(ContractModeBlock){ContractBlockType=ContractModeBlock}
      mask init:
      | set_param(gcb, 'LinkStatus', 'none');
      mask DialogControl DescTextVar Prompt: Mode block
  validator : M-S-Function  LoadFcn=saveValidatorParameters(gcb);  InitFcn=contractBeforeSimulation();  StopFcn=contractAfterSimulation();  FunctionName=contract  mask(ContractValidatorBlock){assumePorts=1, guaranteePorts=4, modePorts=3, ContractBlockType=ContractValidatorBlock, createInportsCheckbox=off}
      mask prompts: assumePorts "Assume ports     :"; guaranteePorts "Guarantee ports :"; modePorts "Mode ports        :"; createInportsCheckbox "Create inports and connect them automatically"
      mask init:
      | set_param(gcb,'LinkStatus','none');
      | contract_callback('inputs_callback',gcb);
      mask DialogControl DescTextVar Prompt: The validator block implements the following logic: <br> <br> <b>Sofar</b>(assume<sub>1</sub> <b>&#8743;</b> assume<sub>2</sub> <b>&#8743;</b> ... assume<sub>k</sub>) <b>&rarr;</b> (guarantee<sub>1</sub> <b>&#8743;</b> guarantee<sub>2</sub> <b>&#8743;</b> ... guarantee<sub>m</sub> <b>&#8743;</b>  mode<sub>1</sub> <b>&#8743;</b> mode<sub>2</sub> <b>&#8743;</b> ... <b>&#8743;</b> mode<sub>n</sub> )<br> where mode<sub>i</sub> = require<sub>i</sub> <b>&rarr;</b> ensure<sub>i</sub>
      mask Display:
      | color('black');
      | port_label('input',1,'assume');
      | port_label('input',2,'guarantee');
      | port_label('input',3,'guarantee');
      | port_label('input',4,'guarantee');
      | port_label('input',5,'guarantee');
      | port_label('input',6,'mode');
      | port_label('input',7,'mode');
      | port_label('input',8,'mode');
      | port_label('output',1,'valid');
  valid : Outport
  wires:
  validator/1 -> Scope/1, valid/1
  population0/1 -> initialPopulation/1(input)
  population/1 -> prepopulation/1, ensure1/1(population), ensure3/1(population), ensure2/1(population), guarantee4/1(population), guarantee1/1(population), guaranteepopulation_gt_0/1(population), guarantee3/1(population)
  require1prePopulation_lt_environmentCapacity/1(require) -> increasing/1(require)
  ensure1/1(ensure) -> increasing/2(ensure)
  require2prePopulation_gt_environmentCapacity/1(require) -> decreasing/1(require)
  ensure2/1(ensure) -> decreasing/2(ensure)
  require3prePopulation_equal_environmentCapacity/1(require) -> stable/1(require)
  ensure3/1(ensure) -> stable/2(ensure)
  environmentCapacity/1 -> require3prePopulation_equal_environmentCapacity/1(environmentCapacity), require2prePopulation_gt_environmentCapacity/1(environmentCapacity), require1prePopulation_lt_environmentCapacity/1(environmentCapacity), guarantee4/2(environmentCapacity), guarantee3/2(environmentCapacity)
  initialPopulation/1(output) -> assumeinitialPopulation_gt_0/1(initialPopulation), guarantee1/2(initialPopulation)
  assumeinitialPopulation_gt_0/1(assume) -> validator/1
  guaranteepopulation_gt_0/1(guarantee) -> validator/2
  guarantee1/1(guarantee) -> validator/3
  guarantee3/1(guarantee) -> validator/4
  increasing/1(mode) -> validator/6
  decreasing/1(mode) -> validator/7
  stable/1(mode) -> validator/8
  guarantee4/1(guarantee) -> validator/5
  prepopulation/1 -> require1prePopulation_lt_environmentCapacity/2(prePopulation), require2prePopulation_gt_environmentCapacity/2(prePopulation), require3prePopulation_equal_environmentCapacity/2(prePopulation)

== system graphicalFun1/bacteriaPopulationSpec/assumeinitialPopulation_gt_0 ==
  initialPopulation : Inport
  CompareToZero : Subsystem  AncestorBlock=|  TreatAsAtomicUnit=on  mask(Compare To Zero){relop=>, OutDataTypeStr=boolean, ZeroCross=on}
      | simulink/Logic and Bit
      | Operations/Compare
      | To Zero
      mask prompts: relop "Simulink:masks:Operator_MP"; OutDataTypeStr "Simulink:masks:OutputDataType_MP"; ZeroCross "Simulink:masks:EnableZerocrossingDetection_MP"
      mask help: Simulink:masks:CompareToZero_MD
      mask init:
      | blkName = gcb;
      | 
      | if strcmp(get_param(gcbh,'OutDataTypeStr'),'boolean')
      | 	setValue = 'boolean';
      | else
      |     setValue = 'fixdt(0, 8)';
      | end
      | 
      | set_param([blkName,'/Compare'],'relop',relop, ...
      | 	'OutDataTypeStr', setValue, 'ZeroCross', ZeroCross);
      mask TypeOptions relop: == | ~= | < | <= | >= | >
      mask TypeOptions OutDataTypeStr: Simulink:masks:uint8 | Simulink:masks:boolean
      mask Callback ZeroCross: sl('zeroCrossEnable', gcbh);
      mask Display: disp([relop,' 0'])
  assume : Outport  OutDataTypeStr=boolean
  wires:
  initialPopulation/1 -> CompareToZero/1(u)
  CompareToZero/1(y) -> assume/1

== system graphicalFun1/bacteriaPopulationSpec/decreasing ==
  note: Shouldn't not be edited
  require : Inport  OutDataTypeStr=boolean
  ensure : Inport  Port=2  OutDataTypeStr=boolean
  and : Logic  Operator=NOT  IconShape=distinctive  AllPortsSameDT=off  OutDataTypeStr=boolean
  or : Logic  Operator=OR  IconShape=distinctive  AllPortsSameDT=off  OutDataTypeStr=boolean
  mode : Outport
  wires:
  require/1 -> and/1
  ensure/1 -> or/2
  and/1 -> or/1
  or/1 -> mode/1

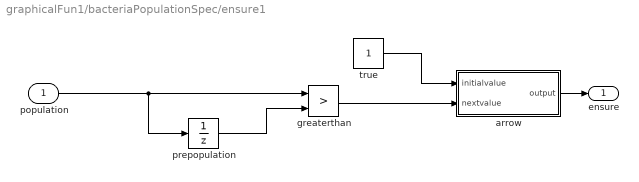
== system graphicalFun1/bacteriaPopulationSpec/ensure1 ==
  population : Inport
  arrow : Subsystem  TreatAsAtomicUnit=on  mask(ArrowOperator){LustreOperatorBlock=ArrowOperator}
      mask prompts: LustreOperatorBlock "ArrowOperator"
  greaterthan : RelationalOperator  Operator=>  OutDataTypeStr=boolean  RndMeth=Nearest
  prepopulation : UnitDelay  SampleTime=-1
  true : Constant  OutDataTypeStr=boolean
  ensure : Outport  OutDataTypeStr=boolean
  wires:
  prepopulation/1 -> greaterthan/2
  true/1 -> arrow/1(initialvalue)
  greaterthan/1 -> arrow/2(nextvalue)
  arrow/1(output) -> ensure/1
  population/1 -> prepopulation/1, greaterthan/1

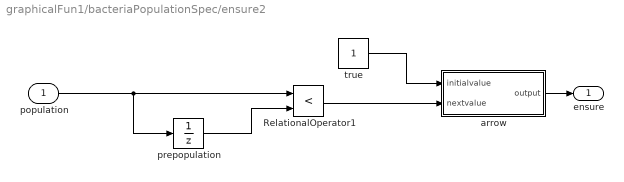
== system graphicalFun1/bacteriaPopulationSpec/ensure2 ==
  population : Inport
  RelationalOperator1 : RelationalOperator  Operator=<  OutDataTypeStr=boolean  RndMeth=Nearest
  arrow : Subsystem  TreatAsAtomicUnit=on  mask(ArrowOperator){LustreOperatorBlock=ArrowOperator}
      mask prompts: LustreOperatorBlock "ArrowOperator"
  prepopulation : UnitDelay  SampleTime=-1
  true : Constant  OutDataTypeStr=boolean
  ensure : Outport  OutDataTypeStr=boolean
  wires:
  prepopulation/1 -> RelationalOperator1/2
  true/1 -> arrow/1(initialvalue)
  RelationalOperator1/1 -> arrow/2(nextvalue)
  arrow/1(output) -> ensure/1
  population/1 -> prepopulation/1, RelationalOperator1/1

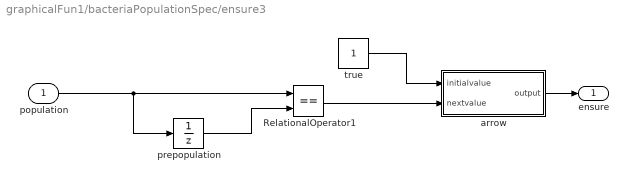
== system graphicalFun1/bacteriaPopulationSpec/ensure3 ==
  population : Inport
  RelationalOperator1 : RelationalOperator  Operator===  OutDataTypeStr=boolean  RndMeth=Nearest
  arrow : Subsystem  TreatAsAtomicUnit=on  mask(ArrowOperator){LustreOperatorBlock=ArrowOperator}
      mask prompts: LustreOperatorBlock "ArrowOperator"
  prepopulation : UnitDelay  SampleTime=-1
  true : Constant  OutDataTypeStr=boolean
  ensure : Outport  OutDataTypeStr=boolean
  wires:
  RelationalOperator1/1 -> arrow/2(nextvalue)
  true/1 -> arrow/1(initialvalue)
  arrow/1(output) -> ensure/1
  population/1 -> prepopulation/1, RelationalOperator1/1
  prepopulation/1 -> RelationalOperator1/2

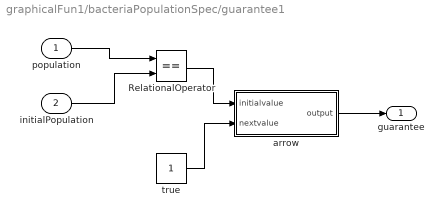
== system graphicalFun1/bacteriaPopulationSpec/guarantee1 ==
  population : Inport
  initialPopulation : Inport  Port=2
  RelationalOperator : RelationalOperator  Operator===  OutDataTypeStr=boolean  RndMeth=Nearest
  arrow : Subsystem  TreatAsAtomicUnit=on  mask(ArrowOperator){LustreOperatorBlock=ArrowOperator}
      mask prompts: LustreOperatorBlock "ArrowOperator"
  true : Constant  OutDataTypeStr=boolean
  guarantee : Outport  OutDataTypeStr=boolean
  wires:
  arrow/1(output) -> guarantee/1
  true/1 -> arrow/2(nextvalue)
  population/1 -> RelationalOperator/1
  initialPopulation/1 -> RelationalOperator/2
  RelationalOperator/1 -> arrow/1(initialvalue)

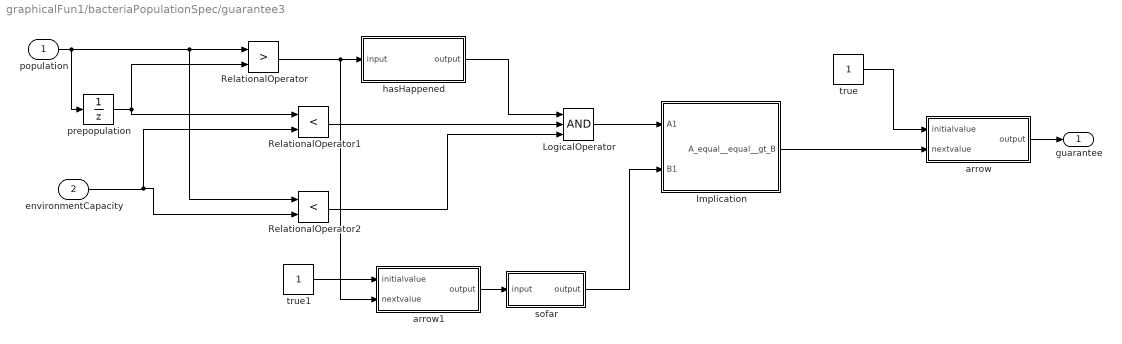
== system graphicalFun1/bacteriaPopulationSpec/guarantee3 ==
  population : Inport
  environmentCapacity : Inport  Port=2
  Implication : Subsystem  TreatAsAtomicUnit=on  mask(CoCoSim-Implies){}
      mask help: CoCoSim block for Logical Implication
      mask Display: disp(' ')
  LogicalOperator : Logic  Inputs=3  AllPortsSameDT=off  OutDataTypeStr=boolean
  RelationalOperator : RelationalOperator  Operator=>  OutDataTypeStr=boolean  RndMeth=Nearest
  RelationalOperator1 : RelationalOperator  Operator=<  OutDataTypeStr=boolean  RndMeth=Nearest
  RelationalOperator2 : RelationalOperator  Operator=<  OutDataTypeStr=boolean  RndMeth=Nearest
  arrow : Subsystem  TreatAsAtomicUnit=on  mask(ArrowOperator){LustreOperatorBlock=ArrowOperator}
      mask prompts: LustreOperatorBlock "ArrowOperator"
  arrow1 : Subsystem  TreatAsAtomicUnit=on  mask(ArrowOperator){LustreOperatorBlock=ArrowOperator}
      mask prompts: LustreOperatorBlock "ArrowOperator"
  hasHappened : Subsystem  TreatAsAtomicUnit=on
  prepopulation : UnitDelay  SampleTime=-1
  sofar : Subsystem  TreatAsAtomicUnit=on
  true : Constant  OutDataTypeStr=boolean
  true1 : Constant  OutDataTypeStr=boolean
  guarantee : Outport  OutDataTypeStr=boolean
  wires:
  population/1 -> prepopulation/1, RelationalOperator2/1, RelationalOperator/1
  prepopulation/1 -> RelationalOperator1/1, RelationalOperator/2
  RelationalOperator/1 -> arrow1/2(nextvalue), hasHappened/1(input)
  hasHappened/1(output) -> LogicalOperator/1
  environmentCapacity/1 -> RelationalOperator2/2, RelationalOperator1/2
  arrow/1(output) -> guarantee/1
  RelationalOperator1/1 -> LogicalOperator/2
  RelationalOperator2/1 -> LogicalOperator/3
  true/1 -> arrow/1(initialvalue)
  true1/1 -> arrow1/1(initialvalue)
  LogicalOperator/1 -> Implication/1(A1)
  sofar/1(output) -> Implication/2(B1)
  arrow1/1(output) -> sofar/1(input)
  Implication/1(A_equal__equal__gt_B) -> arrow/2(nextvalue)

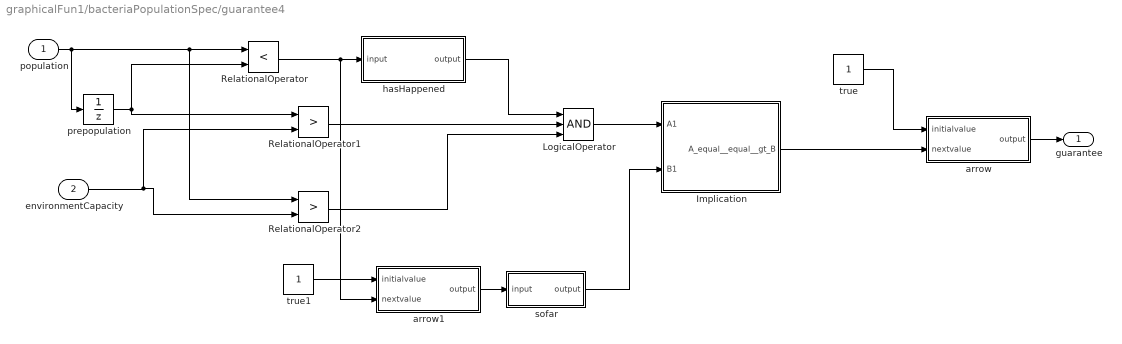
== system graphicalFun1/bacteriaPopulationSpec/guarantee4 ==
  population : Inport
  environmentCapacity : Inport  Port=2
  Implication : Subsystem  TreatAsAtomicUnit=on  mask(CoCoSim-Implies){}
      mask help: CoCoSim block for Logical Implication
      mask Display: disp(' ')
  LogicalOperator : Logic  Inputs=3  AllPortsSameDT=off  OutDataTypeStr=boolean
  RelationalOperator : RelationalOperator  Operator=<  OutDataTypeStr=boolean  RndMeth=Nearest
  RelationalOperator1 : RelationalOperator  Operator=>  OutDataTypeStr=boolean  RndMeth=Nearest
  RelationalOperator2 : RelationalOperator  Operator=>  OutDataTypeStr=boolean  RndMeth=Nearest
  arrow : Subsystem  TreatAsAtomicUnit=on  mask(ArrowOperator){LustreOperatorBlock=ArrowOperator}
      mask prompts: LustreOperatorBlock "ArrowOperator"
  arrow1 : Subsystem  TreatAsAtomicUnit=on  mask(ArrowOperator){LustreOperatorBlock=ArrowOperator}
      mask prompts: LustreOperatorBlock "ArrowOperator"
  hasHappened : Subsystem  TreatAsAtomicUnit=on
  prepopulation : UnitDelay  SampleTime=-1
  sofar : Subsystem  TreatAsAtomicUnit=on
  true : Constant  OutDataTypeStr=boolean
  true1 : Constant  OutDataTypeStr=boolean
  guarantee : Outport  OutDataTypeStr=boolean
  wires:
  RelationalOperator2/1 -> LogicalOperator/3
  Implication/1(A_equal__equal__gt_B) -> arrow/2(nextvalue)
  true/1 -> arrow/1(initialvalue)
  environmentCapacity/1 -> RelationalOperator2/2, RelationalOperator1/2
  sofar/1(output) -> Implication/2(B1)
  RelationalOperator/1 -> arrow1/2(nextvalue), hasHappened/1(input)
  arrow1/1(output) -> sofar/1(input)
  population/1 -> prepopulation/1, RelationalOperator2/1, RelationalOperator/1
  prepopulation/1 -> RelationalOperator1/1, RelationalOperator/2
  arrow/1(output) -> guarantee/1
  RelationalOperator1/1 -> LogicalOperator/2
  LogicalOperator/1 -> Implication/1(A1)
  true1/1 -> arrow1/1(initialvalue)
  hasHappened/1(output) -> LogicalOperator/1

== system graphicalFun1/bacteriaPopulationSpec/guaranteepopulation_gt_0 ==
  population : Inport
  CompareToZero1 : Subsystem  AncestorBlock=|  TreatAsAtomicUnit=on  mask(Compare To Zero){relop=>, OutDataTypeStr=boolean, ZeroCross=on}
      | simulink/Logic and Bit
      | Operations/Compare
      | To Zero
      mask prompts: relop "Simulink:masks:Operator_MP"; OutDataTypeStr "Simulink:masks:OutputDataType_MP"; ZeroCross "Simulink:masks:EnableZerocrossingDetection_MP"
      mask help: Simulink:masks:CompareToZero_MD
      mask init: same as graphicalFun1/bacteriaPopulationSpec/assumeinitialPopulation_gt_0/CompareToZero
      mask TypeOptions relop: == | ~= | < | <= | >= | >
      mask TypeOptions OutDataTypeStr: Simulink:masks:uint8 | Simulink:masks:boolean
      mask Callback ZeroCross: sl('zeroCrossEnable', gcbh);
      mask Display: disp([relop,' 0'])
  guarantee : Outport  OutDataTypeStr=boolean
  wires:
  population/1 -> CompareToZero1/1(u)
  CompareToZero1/1(y) -> guarantee/1

== system graphicalFun1/bacteriaPopulationSpec/increasing ==
  note: Shouldn't not be edited
  require : Inport  OutDataTypeStr=boolean
  ensure : Inport  Port=2  OutDataTypeStr=boolean
  and : Logic  Operator=NOT  IconShape=distinctive  AllPortsSameDT=off  OutDataTypeStr=boolean
  or : Logic  Operator=OR  IconShape=distinctive  AllPortsSameDT=off  OutDataTypeStr=boolean
  mode : Outport
  wires:
  require/1 -> and/1
  ensure/1 -> or/2
  and/1 -> or/1
  or/1 -> mode/1

== system graphicalFun1/bacteriaPopulationSpec/initialPopulation ==
  input : Inport
  arrow : Subsystem  TreatAsAtomicUnit=on  mask(ArrowOperator){LustreOperatorBlock=ArrowOperator}
      mask prompts: LustreOperatorBlock "ArrowOperator"
  preoutput : UnitDelay  InitialCondition=1  SampleTime=-1
  output : Outport
  wires:
  preoutput/1 -> arrow/2(nextvalue)
  input/1 -> arrow/1(initialvalue)
  arrow/1(output) -> output/1, preoutput/1

== system graphicalFun1/bacteriaPopulationSpec/require1prePopulation_lt_environmentCapacity ==
  environmentCapacity : Inport
  prePopulation : Inport  Port=2
  RelationalOperator : RelationalOperator  Operator=<  OutDataTypeStr=boolean  RndMeth=Nearest
  require : Outport  OutDataTypeStr=boolean
  wires:
  prePopulation/1 -> RelationalOperator/1
  environmentCapacity/1 -> RelationalOperator/2
  RelationalOperator/1 -> require/1

== system graphicalFun1/bacteriaPopulationSpec/require2prePopulation_gt_environmentCapacity ==
  environmentCapacity : Inport
  prePopulation : Inport  Port=2
  RelationalOperator : RelationalOperator  Operator=>  OutDataTypeStr=boolean  RndMeth=Nearest
  require : Outport  OutDataTypeStr=boolean
  wires:
  prePopulation/1 -> RelationalOperator/1
  RelationalOperator/1 -> require/1
  environmentCapacity/1 -> RelationalOperator/2

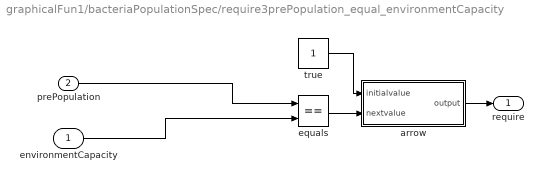
== system graphicalFun1/bacteriaPopulationSpec/require3prePopulation_equal_environmentCapacity ==
  environmentCapacity : Inport
  prePopulation : Inport  Port=2
  arrow : Subsystem  TreatAsAtomicUnit=on  mask(ArrowOperator){LustreOperatorBlock=ArrowOperator}
      mask prompts: LustreOperatorBlock "ArrowOperator"
  equals : RelationalOperator  Operator===  OutDataTypeStr=boolean  RndMeth=Nearest
  true : Constant  OutDataTypeStr=boolean
  require : Outport  OutDataTypeStr=boolean
  wires:
  environmentCapacity/1 -> equals/2
  prePopulation/1 -> equals/1
  true/1 -> arrow/1(initialvalue)
  equals/1 -> arrow/2(nextvalue)
  arrow/1(output) -> require/1

== system graphicalFun1/bacteriaPopulationSpec/stable ==
  note: Shouldn't not be edited
  require : Inport  OutDataTypeStr=boolean
  ensure : Inport  Port=2  OutDataTypeStr=boolean
  and : Logic  Operator=NOT  IconShape=distinctive  AllPortsSameDT=off  OutDataTypeStr=boolean
  or : Logic  Operator=OR  IconShape=distinctive  AllPortsSameDT=off  OutDataTypeStr=boolean
  mode : Outport
  wires:
  require/1 -> and/1
  ensure/1 -> or/2
  and/1 -> or/1
  or/1 -> mode/1

== system graphicalFun1/bacteriaPopulationSpec/assumeinitialPopulation_gt_0/CompareToZero ==
  u : Inport
  Compare : RelationalOperator  Operator=>  OutDataTypeStr=boolean  RndMeth=Nearest  InputSameDT=on
  Constant : Constant  DisableCoverage=on  Value=0  OutDataTypeStr=Inherit: Inherit via back propagation  PreserveConstantTs=on
  y : Outport
  wires:
  Constant/1 -> Compare/2
  u/1 -> Compare/1
  Compare/1 -> y/1

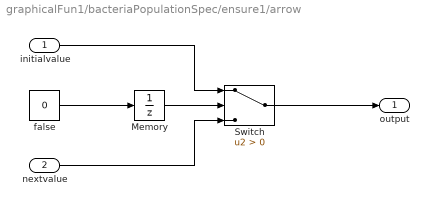
== system graphicalFun1/bacteriaPopulationSpec/ensure1/arrow ==
  initialvalue : Inport
  nextvalue : Inport  Port=2
  Memory : UnitDelay  InitialCondition=1  SampleTime=-1
  Switch : Switch  Criteria=u2 > Threshold
  false : Constant  Value=0  OutDataTypeStr=boolean
  output : Outport
  wires:
  initialvalue/1 -> Switch/1
  false/1 -> Memory/1
  Memory/1 -> Switch/2
  nextvalue/1 -> Switch/3
  Switch/1 -> output/1

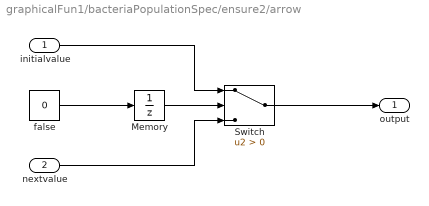
== system graphicalFun1/bacteriaPopulationSpec/ensure2/arrow ==
  initialvalue : Inport
  nextvalue : Inport  Port=2
  Memory : UnitDelay  InitialCondition=1  SampleTime=-1
  Switch : Switch  Criteria=u2 > Threshold
  false : Constant  Value=0  OutDataTypeStr=boolean
  output : Outport
  wires:
  initialvalue/1 -> Switch/1
  false/1 -> Memory/1
  Memory/1 -> Switch/2
  nextvalue/1 -> Switch/3
  Switch/1 -> output/1

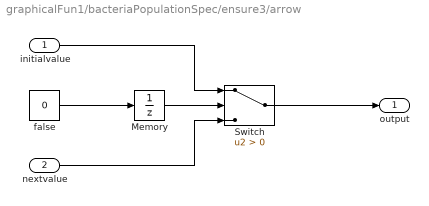
== system graphicalFun1/bacteriaPopulationSpec/ensure3/arrow ==
  initialvalue : Inport
  nextvalue : Inport  Port=2
  Memory : UnitDelay  InitialCondition=1  SampleTime=-1
  Switch : Switch  Criteria=u2 > Threshold
  false : Constant  Value=0  OutDataTypeStr=boolean
  output : Outport
  wires:
  initialvalue/1 -> Switch/1
  false/1 -> Memory/1
  Memory/1 -> Switch/2
  nextvalue/1 -> Switch/3
  Switch/1 -> output/1

== system graphicalFun1/bacteriaPopulationSpec/guarantee1/arrow ==
  initialvalue : Inport
  nextvalue : Inport  Port=2
  Memory : UnitDelay  InitialCondition=1  SampleTime=-1
  Switch : Switch  Criteria=u2 > Threshold
  false : Constant  Value=0  OutDataTypeStr=boolean
  output : Outport
  wires:
  initialvalue/1 -> Switch/1
  false/1 -> Memory/1
  Memory/1 -> Switch/2
  nextvalue/1 -> Switch/3
  Switch/1 -> output/1

== system graphicalFun1/bacteriaPopulationSpec/guarantee3/Implication ==
  A1 : Inport
  B1 : Inport  Port=2
  LogicalOperator : Logic  Operator=OR  AllPortsSameDT=off  OutDataTypeStr=boolean
  LogicalOperator1 : Logic  Operator=NOT  AllPortsSameDT=off  OutDataTypeStr=boolean
  A_equal__equal__gt_B : Outport
  wires:
  A1/1 -> LogicalOperator1/1
  LogicalOperator1/1 -> LogicalOperator/1
  B1/1 -> LogicalOperator/2
  LogicalOperator/1 -> A_equal__equal__gt_B/1

== system graphicalFun1/bacteriaPopulationSpec/guarantee3/arrow ==
  initialvalue : Inport
  nextvalue : Inport  Port=2
  Memory : UnitDelay  InitialCondition=1  SampleTime=-1
  Switch : Switch  Criteria=u2 > Threshold
  false : Constant  Value=0  OutDataTypeStr=boolean
  output : Outport
  wires:
  initialvalue/1 -> Switch/1
  false/1 -> Memory/1
  Memory/1 -> Switch/2
  nextvalue/1 -> Switch/3
  Switch/1 -> output/1

== system graphicalFun1/bacteriaPopulationSpec/guarantee3/arrow1 ==
  initialvalue : Inport
  nextvalue : Inport  Port=2
  Memory : UnitDelay  InitialCondition=1  SampleTime=-1
  Switch : Switch  Criteria=u2 > Threshold
  false : Constant  Value=0  OutDataTypeStr=boolean
  output : Outport
  wires:
  initialvalue/1 -> Switch/1
  false/1 -> Memory/1
  Memory/1 -> Switch/2
  nextvalue/1 -> Switch/3
  Switch/1 -> output/1

== system graphicalFun1/bacteriaPopulationSpec/guarantee3/hasHappened ==
  input : Inport  OutDataTypeStr=boolean
  arrow : Subsystem  TreatAsAtomicUnit=on  mask(ArrowOperator){LustreOperatorBlock=ArrowOperator}
      mask prompts: LustreOperatorBlock "ArrowOperator"
  false : Constant  Value=0  OutDataTypeStr=boolean
  or : Logic  Operator=OR  IconShape=distinctive  AllPortsSameDT=off  OutDataTypeStr=boolean
  preoutput : UnitDelay  InitialCondition=1  SampleTime=-1
  output : Outport  OutDataTypeStr=boolean
  wires:
  arrow/1(output) -> or/2
  or/1 -> preoutput/1, output/1
  false/1 -> arrow/1(initialvalue)
  input/1 -> or/1
  preoutput/1 -> arrow/2(nextvalue)

== system graphicalFun1/bacteriaPopulationSpec/guarantee3/sofar ==
  input : Inport  OutDataTypeStr=boolean
  and : Logic  IconShape=distinctive  AllPortsSameDT=off  OutDataTypeStr=boolean
  arrow : Subsystem  TreatAsAtomicUnit=on  mask(ArrowOperator){LustreOperatorBlock=ArrowOperator}
      mask prompts: LustreOperatorBlock "ArrowOperator"
  preoutput : UnitDelay  InitialCondition=1  SampleTime=-1
  output : Outport  OutDataTypeStr=boolean
  wires:
  preoutput/1 -> and/2
  and/1 -> arrow/2(nextvalue)
  arrow/1(output) -> output/1, preoutput/1
  input/1 -> and/1, arrow/1(initialvalue)

== system graphicalFun1/bacteriaPopulationSpec/guarantee4/Implication ==
  A1 : Inport
  B1 : Inport  Port=2
  LogicalOperator : Logic  Operator=OR  AllPortsSameDT=off  OutDataTypeStr=boolean
  LogicalOperator1 : Logic  Operator=NOT  AllPortsSameDT=off  OutDataTypeStr=boolean
  A_equal__equal__gt_B : Outport
  wires:
  A1/1 -> LogicalOperator1/1
  LogicalOperator1/1 -> LogicalOperator/1
  B1/1 -> LogicalOperator/2
  LogicalOperator/1 -> A_equal__equal__gt_B/1

== system graphicalFun1/bacteriaPopulationSpec/guarantee4/arrow ==
  initialvalue : Inport
  nextvalue : Inport  Port=2
  Memory : UnitDelay  InitialCondition=1  SampleTime=-1
  Switch : Switch  Criteria=u2 > Threshold
  false : Constant  Value=0  OutDataTypeStr=boolean
  output : Outport
  wires:
  initialvalue/1 -> Switch/1
  false/1 -> Memory/1
  Memory/1 -> Switch/2
  nextvalue/1 -> Switch/3
  Switch/1 -> output/1

== system graphicalFun1/bacteriaPopulationSpec/guarantee4/arrow1 ==
  initialvalue : Inport
  nextvalue : Inport  Port=2
  Memory : UnitDelay  InitialCondition=1  SampleTime=-1
  Switch : Switch  Criteria=u2 > Threshold
  false : Constant  Value=0  OutDataTypeStr=boolean
  output : Outport
  wires:
  initialvalue/1 -> Switch/1
  false/1 -> Memory/1
  Memory/1 -> Switch/2
  nextvalue/1 -> Switch/3
  Switch/1 -> output/1

== system graphicalFun1/bacteriaPopulationSpec/guarantee4/hasHappened ==
  input : Inport  OutDataTypeStr=boolean
  arrow : Subsystem  TreatAsAtomicUnit=on  mask(ArrowOperator){LustreOperatorBlock=ArrowOperator}
      mask prompts: LustreOperatorBlock "ArrowOperator"
  false : Constant  Value=0  OutDataTypeStr=boolean
  or : Logic  Operator=OR  IconShape=distinctive  AllPortsSameDT=off  OutDataTypeStr=boolean
  preoutput : UnitDelay  InitialCondition=1  SampleTime=-1
  output : Outport  OutDataTypeStr=boolean
  wires:
  arrow/1(output) -> or/2
  or/1 -> preoutput/1, output/1
  false/1 -> arrow/1(initialvalue)
  input/1 -> or/1
  preoutput/1 -> arrow/2(nextvalue)

== system graphicalFun1/bacteriaPopulationSpec/guarantee4/sofar ==
  input : Inport  OutDataTypeStr=boolean
  and : Logic  IconShape=distinctive  AllPortsSameDT=off  OutDataTypeStr=boolean
  arrow : Subsystem  TreatAsAtomicUnit=on  mask(ArrowOperator){LustreOperatorBlock=ArrowOperator}
      mask prompts: LustreOperatorBlock "ArrowOperator"
  preoutput : UnitDelay  InitialCondition=1  SampleTime=-1
  output : Outport  OutDataTypeStr=boolean
  wires:
  preoutput/1 -> and/2
  and/1 -> arrow/2(nextvalue)
  arrow/1(output) -> output/1, preoutput/1
  input/1 -> and/1, arrow/1(initialvalue)

== system graphicalFun1/bacteriaPopulationSpec/guaranteepopulation_gt_0/CompareToZero1 ==
  u : Inport
  Compare : RelationalOperator  Operator=>  OutDataTypeStr=boolean  RndMeth=Nearest  InputSameDT=on
  Constant : Constant  DisableCoverage=on  Value=0  OutDataTypeStr=Inherit: Inherit via back propagation  PreserveConstantTs=on
  y : Outport
  wires:
  Constant/1 -> Compare/2
  u/1 -> Compare/1
  Compare/1 -> y/1

== system graphicalFun1/bacteriaPopulationSpec/initialPopulation/arrow ==
  initialvalue : Inport
  nextvalue : Inport  Port=2
  Memory : UnitDelay  InitialCondition=1  SampleTime=-1
  Switch : Switch  Criteria=u2 > Threshold
  false : Constant  Value=0  OutDataTypeStr=boolean
  output : Outport
  wires:
  initialvalue/1 -> Switch/1
  false/1 -> Memory/1
  Memory/1 -> Switch/2
  nextvalue/1 -> Switch/3
  Switch/1 -> output/1

== system graphicalFun1/bacteriaPopulationSpec/require3prePopulation_equal_environmentCapacity/arrow ==
  initialvalue : Inport
  nextvalue : Inport  Port=2
  Memory : UnitDelay  InitialCondition=1  SampleTime=-1
  Switch : Switch  Criteria=u2 > Threshold
  false : Constant  Value=0  OutDataTypeStr=boolean
  output : Outport
  wires:
  initialvalue/1 -> Switch/1
  false/1 -> Memory/1
  Memory/1 -> Switch/2
  nextvalue/1 -> Switch/3
  Switch/1 -> output/1

== system graphicalFun1/bacteriaPopulationSpec/guarantee3/hasHappened/arrow ==
  initialvalue : Inport
  nextvalue : Inport  Port=2
  Memory : UnitDelay  InitialCondition=1  SampleTime=-1
  Switch : Switch  Criteria=u2 > Threshold
  false : Constant  Value=0  OutDataTypeStr=boolean
  output : Outport
  wires:
  initialvalue/1 -> Switch/1
  false/1 -> Memory/1
  Memory/1 -> Switch/2
  nextvalue/1 -> Switch/3
  Switch/1 -> output/1

== system graphicalFun1/bacteriaPopulationSpec/guarantee3/sofar/arrow ==
  initialvalue : Inport
  nextvalue : Inport  Port=2
  Memory : UnitDelay  InitialCondition=1  SampleTime=-1
  Switch : Switch  Criteria=u2 > Threshold
  false : Constant  Value=0  OutDataTypeStr=boolean
  output : Outport
  wires:
  initialvalue/1 -> Switch/1
  false/1 -> Memory/1
  Memory/1 -> Switch/2
  nextvalue/1 -> Switch/3
  Switch/1 -> output/1

== system graphicalFun1/bacteriaPopulationSpec/guarantee4/hasHappened/arrow ==
  initialvalue : Inport
  nextvalue : Inport  Port=2
  Memory : UnitDelay  InitialCondition=1  SampleTime=-1
  Switch : Switch  Criteria=u2 > Threshold
  false : Constant  Value=0  OutDataTypeStr=boolean
  output : Outport
  wires:
  initialvalue/1 -> Switch/1
  false/1 -> Memory/1
  Memory/1 -> Switch/2
  nextvalue/1 -> Switch/3
  Switch/1 -> output/1

== system graphicalFun1/bacteriaPopulationSpec/guarantee4/sofar/arrow ==
  initialvalue : Inport
  nextvalue : Inport  Port=2
  Memory : UnitDelay  InitialCondition=1  SampleTime=-1
  Switch : Switch  Criteria=u2 > Threshold
  false : Constant  Value=0  OutDataTypeStr=boolean
  output : Outport
  wires:
  initialvalue/1 -> Switch/1
  false/1 -> Memory/1
  Memory/1 -> Switch/2
  nextvalue/1 -> Switch/3
  Switch/1 -> output/1

== stateflow chart graphicalFun1/bacteriaPopulation/bacteriaPopulation ==
  state [x1, y1] = gupdate(x,y) [function]
    (default) -> (junction 104)
    (junction 104) -> (junction 110) [order 2] : [ y < 32.0 ]{x1 = y; y1 = y*2;}
    (junction 104) -> (junction 111) [order 1]
    (junction 111) -> (junction 110) [order 1] : [ y > 32.0 ]{x1 = y; y1 = y/2;}
    (junction 110) -> (junction 120) : {disp('efefe')}
    (junction 112) -> (junction 110) : {x1 = x; y1 = y;}
    (junction 111) -> (junction 112) [order 2]
  state start
    entry:
    prePopulation = population0;
    population = population0;
  state state
    entry:
    [prePopulation, population] = gupdate(prePopulation, population);
  (default) -> start
  state -> (junction 13)
  start -> (junction 13)
  (junction 13) -> state
  data: x function_input; y function_input; x1 function_output size=1; y1 function_output size=1; population output; population0 input; prePopulation local
  events: dummyEvent local FUNCTION_CALL_EVENT
